simulink model "PhaseII_opalrt_NoProtection"  (Simulink 8.8)
settings: Solver=ode3  StartTime=0.0  StopTime=inf  FixedStep=Ts  RelTol=1e-5  EnableMultiTasking=on
PostLoadFcn:
  | %BESS ctrl
  | Kpf=0.005*3*12;
  | Kif=5*6;
  | 
  | Kpf1=0.005*3*12;
  | Kif1=5*6;
  | Kp_v=0.016*15*35;
  | Ki_v=12*25;
  | 
  | Kp_v1=0.016*15*35;
  | Ki_v1=12*25;
  | 
  | Vabc_B=12.47e3;
  | Vdc_ref=Vabc_B*2;
  | Kpwm=sqrt(2)*Vabc_B/Vdc_ref;
  | ZB=Vabc_B^2/1e6;
  | R=0.005*ZB;
  | Ibasefull=673/2*sqrt(2);
  | 
  | 
  | Ts_Control=1e-4;
  | ts=0.05;
  | delay=0.2;
  | offset=10e3;
  | t_plan=60;
  | t_monitor=.2;
  | t_mon=t_monitor;
  | scalingfactor=1;
  | x=0.5;
  | n=6;
  | %t_plan=1/15;
  | %t_monitor=10/900;
  | %t_mon=10/900;
  | 
  | %t_plan=1/5;
  | %t_monitor=10/300;
  | %t_mon=10/300;
  | %scalingfactor=1/300;
  | 
  | f0=60;
  | 
  | Pabc_B=1e6;
  | Iabc_B=Pabc_B*sqrt(2/3)/Vabc_B;  % pk value
  | Imax_1=2.5;
  | Ptrans_B=Pabc_B*200;
  | 
  | Vdc_ref=Vabc_B*2;
  | 
  | ZB=Vabc_B^2/Pabc_B;
  | L=0.1*ZB/2/pi/60;
  | R=0.1*ZB;
  | C=1/(4*pi^2*(2e3)^2*L);
  | 
  | LL=0.005*ZB/2/pi/60;
  | RR=0.005*ZB;
  | 
  | RC=0.02;
  | 
  | %%% Initial SOC %%%%
  | SOC_ini_BESS1=0.5;
  | ... (+223 lines)
InitFcn:
  | %BESS ctrl
  | Kpf=0.005*3*12;
  | Kif=5*6;
  | 
  | Kpf1=0.005*3*12;
  | Kif1=5*6;
  | Kp_v=0.016*15*35;
  | Ki_v=12*25;
  | 
  | Kp_v1=0.016*15*35;
  | Ki_v1=12*25;
  | 
  | Vabc_B=12.47e3;
  | Vdc_ref=Vabc_B*2;
  | Kpwm=sqrt(2)*Vabc_B/Vdc_ref;
  | ZB=Vabc_B^2/1e6;
  | R=0.005*ZB;
  | Ibasefull=673/2*sqrt(2);
  | 
  | 
  | Ts_Control=1e-4;
  | ts=0.05;
  | delay=0.2;
  | offset=10e3;
  | t_plan=60;
  | t_monitor=.2;
  | t_mon=t_monitor;
  | scalingfactor=1;
  | x=0.5;
  | n=6;
  | %t_plan=1/15;
  | %t_monitor=10/900;
  | %t_mon=10/900;
  | 
  | %t_plan=1/5;
  | %t_monitor=10/300;
  | %t_mon=10/300;
  | %scalingfactor=1/300;
  | 
  | f0=60;
  | 
  | Pabc_B=1e6;
  | Iabc_B=Pabc_B*sqrt(2/3)/Vabc_B;  % pk value
  | Imax_1=2.5;
  | Ptrans_B=Pabc_B*200;
  | 
  | Vdc_ref=Vabc_B*2;
  | 
  | ZB=Vabc_B^2/Pabc_B;
  | L=0.1*ZB/2/pi/60;
  | R=0.1*ZB;
  | C=1/(4*pi^2*(2e3)^2*L);
  | 
  | LL=0.005*ZB/2/pi/60;
  | RR=0.005*ZB;
  | 
  | RC=0.02;
  | 
  | %%% Initial SOC %%%%
  | SOC_ini_BESS1=0.5;
  | ... (+223 lines)
undefined symbols (not defined in the file): D1, Delta, DiscIntNeverNeededParam, Left, PG2ref, type, V
libraries: powerlib x220, powerlib_meascontrol x82, dspstat3 x54, dsparch4 x43, dspswit3 x24, simulink x19, simulink_extras x12, powerlib_extras x11, ssn_lib x7, artemis x6, rtlab x5, rtio_generic_dnp3 x5
(part 3 of 9)

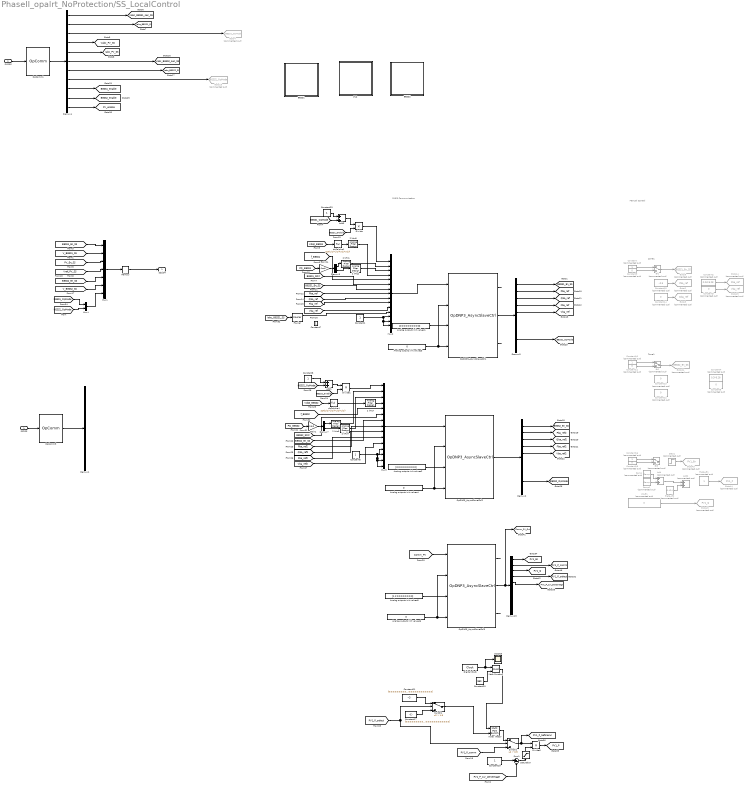
== system PhaseII_opalrt_NoProtection/SS_LocalControl ==
  note: DNP3 Communication
  note: Manual Control
  note: Zone1
  note: Zone1
  SC2SS : Inport
  SM2SS : Inport  Port=2
  2 kHz{1..5,7} (6 alike) : dsparch4/Analog Filter Design  method=Butterworth  filttype=Lowpass  N=2  Wlo=2*pi*5  Whi=80  Rp=2  Rs=40
  Add : Sum  Commented=on
  Add1 : Sum
  Add2 : Sum  Commented=on
  Add3 : Sum
  Analog outputs init values1 : Constant  Value=[0 0 0 0 0 0 0 0 0 0]
  Analog outputs init values2 : Constant  Value=[0 0 0 0 0 0 0 0 0 0]
  Analog outputs init values3 : Constant  Value=0
  Analog outputs init values4 : Constant  Value=0
  Analog outputs init values5 : Constant  Value=[1 2 0 0 0 0 0 0 0 0]
  Analog outputs init values6 : Constant  Value=0
  BESS1 : Subsystem
  BESS2 : Subsystem
  Br1 : ManualSwitch  Commented=on
  Br2 : ManualSwitch  Commented=on
  Br3 : ManualSwitch  Commented=on
  Constant : Constant  Commented=on
  Constant{1,6..8,19,23} (6 alike) : Constant
  Constant10 : Constant  Commented=on
  Constant{3,5,9,11..14,18} (8 alike) : Constant  Commented=on  Value=0
  Constant15 : Constant  Commented=on  Value=-0.5
  Constant16 : Constant  Commented=on
  Constant17 : Constant  Value=[0,0,0,0,0,0,0,0,0,0,0,0,0,0,0,0,0,0,0,0,0,0,0,0,0,0,0,0,0,0,0,0,0,0,0,0,0,0,0,0,0.00637590701003014,0.00637590701003014,0.00637590701003014,0.00637590701003014,0.00637590701003014,0.00637590701003014,0.00637590701003014,0.00637590701003014,0.00637590701003014,0.00637590701003014,0.00637590701003014,0.00637590701003014,0.00637590701003014,0.00637590701003014,0.00637590701003014,0.00637590701003014,0.00637590701003014,0.00637590701003014,0.00637590701003014,0.00637590701003014,0.0597883305113194,0.0597883305113194,0.0597883305113194,0.0597883305113194,0.0597883305113194,0.0597883305113194,0.0597883305113194,0.0597883305113194,0.0597883305113194,0.0597883305113194,0.0597883305113194,0.0597883305113194,0.0597883305113194,0.0597883305113194,0.0597883305113194,0.0597883305113194,0.0597883305113194,0.0597883305113194,0.0597883305113194,0.0597883305113194,0.191640198758314,0.191640198758314,0.191640198758314,0.191640198758314,0.191640198758314,0.191640198758314,0.191640198758314,0.191640198758314,0.191640198758314,0.191640198758314,0.191640198758314,0.191640198758314,0.191640198758314,0.191640198758314,0.191640198758314,0.191640198758314,0.191640198758314,0.191640198758314,0.191640198758314,0.191640198758314,0.258183655928258,0.258183655928258,0.258183655928258,0.258183655928258,0.258183655928258,0.258183655928258,0.258183655928258,0.258183655928258,0.258183655928258,0.258183655928258,0.258183655928258,0.258183655928258,0.258183655928258,0.258183655928258,0.258183655928258,0.258183655928258,0.258183655928258,0.258183655928258,0.258183655928258,0.258183655928258,0.318938480096502,0.318938480096502,0.318938480096502,0.318938480096502,0.318938480096502,0.318938480096502,0.318938480096502,0.318938480096502,0.318938480096502,0.318938480096502,0.318938480096502,0.318938480096502,0.318938480096502,0.318938480096502,0.318938480096502,0.318938480096502,0.318938480096502,0.318938480096502,0.318938480096502,0.318938480096502,0.451835046830676,0.451835046830676,0.451835046830676,0.451835046830676,0.451835046830676,0.451835046830676,0.451835046830676,0.451835046830676,0.451835046830676,0.451835046830676,0.451835046830676,0.451835046830676,0.451835046830676,0.451835046830676,0.451835046830676,0.451835046830676,0.451835046830676,0.451835046830676,0.451835046830676,0.451835046830676,0.659184087530387,0.659184087530387,0.659184087530387,0.659184087530387,0.659184087530387,0.659184087530387,0.659184087530387,0.659184087530387,0.659184087530387,0.659184087530387,0.659184087530387,0.659184087530387,0.659184087530387,0.659184087530387,0.659184087530387,0.659184087530387,0.659184087530387,0.659184087530387,0.659184087530387,0.659184087530387,0.827159209540989,0.827159209540989,0.827159209540989,0.827159209540989,0.827159209540989,0.827159209540989,0.827159209540989,0.827159209540989,0.827159209540989,0.827159209540989,0.827159209540989,0.827159209540989,0.827159209540989,0.827159209540989,0.827159209540989,0.827159209540989,0.827159209540989,0.827159209540989,0.827159209540989,0.827159209540989,1.02022332643508,1.02022332643508,1.02022332643508,1.02022332643508,1.02022332643508,1.02022332643508,1.02022332643508,1.02022332643508,1.02022332643508,1.02022332643508,1.02022332643508,1.02022332643508,1.02022332643508,1.02022332643508,1.02022332643508,1.02022332643508,1.02022332643508,1.02022332643508,1.02022332643508,1.02022332643508,1.18871489543793,1.18871489543793,1.18871489543793,1.18871489543793,1.18871489543793,1.18871489543793,1.18871489543793,1.18871489543793,1.18871489543793,1.18871489543793,1.18871489543793,1.18871489543793,1.18871489543793,1.18871489543793,1.18871489543793,1.18871489543793,1.18871489543793,1.18871489543793,1.18871489543793,1.18871489543793,1.35005293581671,1.35005293581671,1.35005293581671,1.35005293581671,1.35005293581671,1.35005293581671,1.35005293581671,1.35005293581671,1.35005293581671,1.35005293581671,1.35005293581671,1.35005293581671,1.35005293581671,1.35005293581671,1.35005293581671,1.35005293581671,1.35005293581671 ...(+10071 chars)]
  Constant2 : Constant  Commented=on  Value=0.04*6.28
  Constant20 : Constant  Value=960
  Constant21 : Constant  Value=[0,0,0,0,0,0,0,0,0,0,0,0,0,0,0,0,0,0,0,0,0,0,0,0,0,0,0,0,0,0,0,0,0,0,0,0,0,0,0,0,0,0,0,0,0,0,0,0,0,0,0,0,0,0,0,0,0,0,0,0,0.00981250996274463,0.00981250996274463,0.00981250996274463,0.00981250996274463,0.00981250996274463,0.00981250996274463,0.00981250996274463,0.00981250996274463,0.00981250996274463,0.00981250996274463,0.00981250996274463,0.00981250996274463,0.00981250996274463,0.00981250996274463,0.00981250996274463,0.00981250996274463,0.00981250996274463,0.00981250996274463,0.00981250996274463,0.00981250996274463,0.132748194010081,0.132748194010081,0.132748194010081,0.132748194010081,0.132748194010081,0.132748194010081,0.132748194010081,0.132748194010081,0.132748194010081,0.132748194010081,0.132748194010081,0.132748194010081,0.132748194010081,0.132748194010081,0.132748194010081,0.132748194010081,0.132748194010081,0.132748194010081,0.132748194010081,0.132748194010081,0.386564366030885,0.386564366030885,0.386564366030885,0.386564366030885,0.386564366030885,0.386564366030885,0.386564366030885,0.386564366030885,0.386564366030885,0.386564366030885,0.386564366030885,0.386564366030885,0.386564366030885,0.386564366030885,0.386564366030885,0.386564366030885,0.386564366030885,0.386564366030885,0.386564366030885,0.386564366030885,0.625701271422546,0.625701271422546,0.625701271422546,0.625701271422546,0.625701271422546,0.625701271422546,0.625701271422546,0.625701271422546,0.625701271422546,0.625701271422546,0.625701271422546,0.625701271422546,0.625701271422546,0.625701271422546,0.625701271422546,0.625701271422546,0.625701271422546,0.625701271422546,0.625701271422546,0.625701271422546,0.553924369190750,0.553924369190750,0.553924369190750,0.553924369190750,0.553924369190750,0.553924369190750,0.553924369190750,0.553924369190750,0.553924369190750,0.553924369190750,0.553924369190750,0.553924369190750,0.553924369190750,0.553924369190750,0.553924369190750,0.553924369190750,0.553924369190750,0.553924369190750,0.553924369190750,0.553924369190750,0.647873932663837,0.647873932663837,0.647873932663837,0.647873932663837,0.647873932663837,0.647873932663837,0.647873932663837,0.647873932663837,0.647873932663837,0.647873932663837,0.647873932663837,0.647873932663837,0.647873932663837,0.647873932663837,0.647873932663837,0.647873932663837,0.647873932663837,0.647873932663837,0.647873932663837,0.647873932663837,1.50320712211045,1.50320712211045,1.50320712211045,1.50320712211045,1.50320712211045,1.50320712211045,1.50320712211045,1.50320712211045,1.50320712211045,1.50320712211045,1.50320712211045,1.50320712211045,1.50320712211045,1.50320712211045,1.50320712211045,1.50320712211045,1.50320712211045,1.50320712211045,1.50320712211045,1.50320712211045,1.50449928127173,1.50449928127173,1.50449928127173,1.50449928127173,1.50449928127173,1.50449928127173,1.50449928127173,1.50449928127173,1.50449928127173,1.50449928127173,1.50449928127173,1.50449928127173,1.50449928127173,1.50449928127173,1.50449928127173,1.50449928127173,1.50449928127173,1.50449928127173,1.50449928127173,1.50449928127173,2,2,2,2,2,2,2,2,2,2,2,2,2,2,2,2,2,2,2,2,1.59623976041451,1.59623976041451,1.59623976041451,1.59623976041451,1.59623976041451,1.59623976041451,1.59623976041451,1.59623976041451,1.59623976041451,1.59623976041451,1.59623976041451,1.59623976041451,1.59623976041451,1.59623976041451,1.59623976041451,1.59623976041451,1.59623976041451,1.59623976041451,1.59623976041451,1.59623976041451,1.04765330636163,1.04765330636163,1.04765330636163,1.04765330636163,1.04765330636163,1.04765330636163,1.04765330636163,1.04765330636163,1.04765330636163,1.04765330636163,1.04765330636163,1.04765330636163,1.04765330636163,1.04765330636163,1.04765330636163,1.04765330636163,1.04765330636163,1.04765330636163,1.04765330636163,1.04765330636163,0.944545776431073,0.944545776431073,0.944545776431073,0.944545776431073,0.944545776431073,0.944545776431073,0.944545776431073,0.944545776431073,0.944545776431073,0.944545776431073,0.944545776431073,0.944545776431073,0.944545776431073,0.944545776431073,0.944545776431073 ...(+10070 chars)]
  Constant4 : Constant  Commented=on  Value=0.2*6.28
  Demux1 : Demux  Outputs=[1 1 1 1 1 1]
  Demux13 : Demux  Outputs=10
  Demux2 : Demux  Outputs=10
  Demux3 : Demux  Outputs=2
  Demux4 : Demux  Outputs=[3 3 1 3 3 3 3 1 1 1 1]
  Demux5 : Demux  Outputs=10
  Demux7 : Demux  Outputs=2
  Digital Clock : DigitalClock  SampleTime=[0,1]
  Divide : Product  Inputs=**
  Divide1 : Product  Inputs=**
  Divide6 : Product  Inputs=**
  Fourier : powerlib_meascontrol/Measurements/Fourier  Freq=60  n=1  InInit=[0, 0]  Ts=0
  Gain1 : Gain  Gain=-1e-6
  Gain24 : Gain  Gain=-1e-6
  Goto14 : Goto  Commented=on  GotoTag=Fba_ref  TagVisibility=global
  Goto15 : Goto  Commented=on  GotoTag=Vba_ref  TagVisibility=global
  Goto2 : Goto  Commented=on  GotoTag=Pba_ref  TagVisibility=global
  Goto23 : Goto  Commented=on  GotoTag=BESS2_OpMode  TagVisibility=global
  Goto24 : Goto  Commented=on  GotoTag=BESS2_En_SS  TagVisibility=global
  Goto3 : Goto  Commented=on  GotoTag=Qba_ref  TagVisibility=global
  Goto4 : Goto  Commented=on  GotoTag=BESS1_OpMode  TagVisibility=global
  Goto43 : Goto  Commented=on  GotoTag=PV1_En  TagVisibility=global
  Goto44 : Goto  Commented=on  GotoTag=PV1_P  TagVisibility=global
  Goto45 : Goto  Commented=on  GotoTag=PV1_Q  TagVisibility=global
  Goto9 : Goto  Commented=on  GotoTag=BESS1_En_SS  TagVisibility=global
  Index Vector : MultiPortSwitch  DataPortOrder=Zero-based contiguous  Inputs=1  zeroidx=on
  Math Function : Math  Operator=mod  SaturateOnIntegerOverflow=on
  Memory : Memory
  Mux1 : Mux  Inputs=[1 3 1 3 1 3 2]
  Mux2 : Mux  Inputs=15
  Mux3 : Mux  Inputs=15
  Mux4 : Mux  Inputs=2
  OpComm1 : rtlab/OpComm  nbport=1  groupe_acq=1  subsys_rate=0  st=0  Synchronization=on  Interpolation=on  Threshold=1.0  Missed_Data=off  Sim_Time=off  Samples=off  dynSigOut=off  from_console=0  warning_done=off  writeOpCommFile=off  Offset=off
  OpComm3 : rtlab/OpComm  nbport=1  groupe_acq=1  subsys_rate=0  st=0  Synchronization=on  Interpolation=on  Threshold=1.0  Missed_Data=off  Sim_Time=off  Samples=off  dynSigOut=off  from_console=1  warning_done=off  writeOpCommFile=off  Offset=off
  OpDNP3_AsyncSlaveCtrl1 : rtio_generic_dnp3/OpDNP3_AsyncSlaveCtrl  dev_id=3  nbr_aout=10  nbr_bout=1  cfg_name='AsyncDNP3_Slave_cfg.xml'  exe_name='AsyncDNP3_Slave'  nic_name='eth3'  link_addr_remote=7  link_addr_local=8  ip_addr_local='160.36.56.202'  tcp_port_local=18000  dnp3_options=0
  OpDNP3_AsyncSlaveCtrl2 : rtio_generic_dnp3/OpDNP3_AsyncSlaveCtrl  dev_id=4  nbr_aout=10  nbr_bout=1  cfg_name='AsyncDNP3_Slave_cfg.xml'  exe_name='AsyncDNP3_Slave'  nic_name='eth3'  link_addr_remote=9  link_addr_local=10  ip_addr_local='160.36.56.207'  tcp_port_local=18000  dnp3_options=0
  OpDNP3_AsyncSlaveCtrl3 : rtio_generic_dnp3/OpDNP3_AsyncSlaveCtrl  dev_id=2  nbr_aout=10  nbr_bout=1  cfg_name='AsyncDNP3_Slave_cfg.xml'  exe_name='AsyncDNP3_Slave'  nic_name='eth3'  link_addr_remote=5  link_addr_local=6  ip_addr_local='160.36.56.201'  tcp_port_local=18000  dnp3_options=0
  PV2 : Subsystem
  Ramp : simulink/Sources/Ramp  Commented=on  slope=0.5  start=0.5  X0=0
  Ramp1 : simulink/Sources/Ramp  Commented=on  slope=-0.5  start=2.762  X0=0
  Saturation : Saturate  UpperLimit=1  LowerLimit=0
  Scope3 : Scope
  Step1 : Step  Commented=on  SampleTime=0
  Sum1 : Sum  Inputs=|+-
  Switch1 : Switch  Criteria=u2 > Threshold  Threshold=1.5
  Switch2 : Switch  Criteria=u2 > Threshold  Threshold=0.5
  Vd_G1 : Constant  Commented=on  Value=0
  dq2alpha1 : Fcn  Expr=sqrt(u(1)*u(1)+u(2)*u(2))
  dq2alpha4 : Fcn  Expr=sqrt(u(1)*u(1)+u(2)*u(2))
  theta_G1 : Constant  Commented=on
  theta_G2 : Constant  Commented=on  Value=0.424
  "SS2SM " : Outport
  tag scope: BESS1_En_SS=global, BESS1_OpMode=global, BESS1_enable=global, BESS2_En_SS=global, BESS2_OpMode=global, BESS2_enable=global, Comm_PV_Out=global, Fba_ref2=global, Fba_ref=global, Iabc_BESS1_SS=global, Iabc_BESS2_SS=global, Iabc_PV_SS=global, PV1_En=global, PV1_P=global, PV1_P_beforecur=global, PV1_P_comm=global, PV1_P_cur_percentage=global, PV1_P_select=global, PV1_Q=global, PV_enable=global, Pba_ref2=global, Pba_ref=global, Qba_ref2=global, Qba_ref=global, Vabc_BESS1_sec_SS=global, Vabc_BESS2_sec_SS=global, Vabc_PV_SS=global, Vba_ref2=global, Vba_ref=global
  wires:
  SC2SS/1 -> OpComm3/1
  SM2SS/1 -> OpComm1/1
  OpComm1/1 -> Demux4/1
  Demux4/1 -> [Vabc_BESS1_sec_SS]
  Demux4/2 -> [Iabc_BESS1_SS]
  Memory/1 -> "SS2SM "/1
  Mux1/1 -> Memory/1
  [BESS1_En_SS] -> Mux1/1
  [V_BESS1_SS] -> Mux1/2
  OpComm3/1 -> Demux1/1
  Demux4/4 -> [Vabc_PV_SS]
  Demux4/5 -> [Iabc_PV_SS]
  [PV_En_SS] -> Mux1/3
  [Vref_PV_SS] -> Mux1/4
  Constant2/1 -> Goto14/1
  Constant3/1 -> Goto15/1
  [BESS2_En_SS] -> Mux1/5
  [V_BESS2_SS] -> Mux1/6
  Demux4/6 -> [Vabc_BESS2_sec_SS]
  Demux4/7 -> [Iabc_BESS2_SS]
  Demux4/9 -> [BESS1_enable]
  Demux4/10 -> [BESS2_enable]
  Demux4/3 -> Goto4/1
  [BESS1_OpMode] -> Add3/2
  Constant23/1 -> Add3/1
  Add3/1 -> Divide/1
  [BESS1_enable] -> Divide/2
  [Vdq0_BESS1] -> dq2alpha1/1
  Demux3/1 -> 2 kHz1/1
  Demux3/2 -> 2 kHz2/1
  [PQ_BESS1] -> Gain24/1
  Divide/1 -> Mux2/1
  [BESS1_SOC] -> Mux2/6
  Constant1/1 -> Mux2/15, Mux2/14, Mux2/13
  Analog outputs init values3/1 -> OpDNP3_AsyncSlaveCtrl1/2, OpDNP3_AsyncSlaveCtrl1/4
  OpDNP3_AsyncSlaveCtrl1/2 -> Demux5/1
  OpDNP3_AsyncSlaveCtrl1/3 -> ?
  OpDNP3_AsyncSlaveCtrl1/1 -> ?
  Mux2/1 -> OpDNP3_AsyncSlaveCtrl1/1
  Analog outputs init values1/1 -> OpDNP3_AsyncSlaveCtrl1/3
  Demux5/1 -> [BESS1_En_SS]
  Demux5/2 -> [Pba_ref]
  Demux5/3 -> [Qba_ref]
  Demux5/4 -> [Fba_ref]
  Demux5/5 -> [Vba_ref]
  [BESS1_En_SS] -> Mux2/7
  [Pba_ref] -> Mux2/8
  [Qba_ref] -> Mux2/9
  [Fba_ref] -> Mux2/10
  [Vba_ref] -> Mux2/11
  [Iabc_BESS1_SS] -> Fourier/1
  Fourier/1 -> Mux2/12
  Demux4/11 -> [PV_enable]
  [BESS2_OpMode] -> Add1/2
  Constant8/1 -> Add1/1
  Add1/1 -> Divide1/1
  [BESS2_enable] -> Divide1/2
  [Vdq0_BESS2] -> dq2alpha4/1
  Demux7/1 -> 2 kHz3/1
  Demux7/2 -> 2 kHz4/1
  [PQ_BESS2] -> Gain1/1
  Divide1/1 -> Mux3/1
  [BESS2_SOC] -> Mux3/6
  [BESS2_En_SS] -> Mux3/7
  [Pba_ref2] -> Mux3/8
  [Qba_ref2] -> Mux3/9
  [Fba_ref2] -> Mux3/10
  [Vba_ref2] -> Mux3/11
  Constant6/1 -> Mux3/12, Mux3/13, Mux3/14, Mux3/15
  Analog outputs init values4/1 -> OpDNP3_AsyncSlaveCtrl2/4, OpDNP3_AsyncSlaveCtrl2/2
  Analog outputs init values2/1 -> OpDNP3_AsyncSlaveCtrl2/3
  Mux3/1 -> OpDNP3_AsyncSlaveCtrl2/1
  OpDNP3_AsyncSlaveCtrl2/2 -> Demux2/1
  Demux2/1 -> [BESS2_En_SS]
  Demux2/2 -> [Pba_ref2]
  Demux2/3 -> [Qba_ref2]
  Demux2/4 -> [Fba_ref2]
  Demux2/5 -> [Vba_ref2]
  Constant/1 -> Br1/1
  Constant9/1 -> Br1/2
  Constant10/1 -> Br2/1
  Constant11/1 -> Br2/2
  Constant15/1 -> Goto2/1
  Constant14/1 -> Goto3/1
  Analog outputs init values6/1 -> OpDNP3_AsyncSlaveCtrl3/4, OpDNP3_AsyncSlaveCtrl3/2
  OpDNP3_AsyncSlaveCtrl3/2 -> Demux13/1, [Comm_PV_Out]
  OpDNP3_AsyncSlaveCtrl3/3 -> ?
  OpDNP3_AsyncSlaveCtrl3/1 -> ?
  [Comm_PV] -> OpDNP3_AsyncSlaveCtrl3/1
  Demux13/1 -> [PV1_En]
  Demux13/3 -> [PV1_Q]
  Constant16/1 -> Br3/1
  Constant18/1 -> Br3/2
  Vd_G1/1 -> Goto45/1
  Demux13/2 -> [PV1_P_comm]
  Constant20/1 -> Math Function/2
  Math Function/1 -> Index Vector/1
  Constant21/1 -> Switch1/1
  Switch1/1 -> Index Vector/2
  Demux13/4 -> [PV1_P_select]
  Constant17/1 -> Switch1/3
  [PV1_P_select] -> Switch1/2, Switch2/2
  [PV1_P_comm] -> Switch2/3
  Index Vector/1 -> Switch2/1
  Digital Clock/1 -> Scope3/1, Math Function/1
  Demux13/5 -> [PV1_P_cur_percentage]
  Switch2/1 -> [PV1_P_beforecur], Divide6/1
  Divide6/1 -> [PV1_P]
  Constant19/1 -> Sum1/1
  [PV1_P_cur_percentage] -> Sum1/2
  Sum1/1 -> Saturation/1
  Saturation/1 -> Divide6/2
  Analog outputs init values5/1 -> OpDNP3_AsyncSlaveCtrl3/3
  Step1/1 -> Goto43/1
  Ramp/1 -> Add/1
  Ramp1/1 -> Add/2
  Add/1 -> Add2/1
  theta_G2/1 -> Add2/2
  theta_G1/1 -> Goto44/1
  Gain24/1 -> Demux3/1
  Gain1/1 -> Demux7/1
  2 kHz1/1 -> Mux2/2
  2 kHz2/1 -> Mux2/3
  dq2alpha1/1 -> 2 kHz5/1
  [f_BESS1] -> Mux2/5
  dq2alpha4/1 -> 2 kHz7/1
  [f_BESS2] -> Mux3/5
  2 kHz3/1 -> Mux3/2
  2 kHz4/1 -> Mux3/3
  [BESS1_OpMode] -> Mux4/1
  [BESS2_OpMode] -> Mux4/2
  Mux4/1 -> Mux1/7
  Br1/1 -> Goto9/1
  Br2/1 -> Goto24/1
  Demux5/9 -> [BESS1_OpMode]
  Demux2/9 -> [BESS2_OpMode]
  Demux4/8 -> Goto23/1
  2 kHz5/1 -> Mux2/4
  2 kHz7/1 -> Mux3/4

== system PhaseII_opalrt_NoProtection/SM_System/Battery 2 ==
  Demux2 : Demux  Outputs=3
  Gain2 : Gain
  Gain3 : Gain  Gain=Vdc_ref/2
  Gain5 : Gain  Gain=480
  vsa : powerlib/Electrical Sources/Controlled Voltage Source  Initialize=on  Source_Type=AC  Amplitude=0  Phase=0  Frequency=0  Measurements=None
  vsb : powerlib/Electrical Sources/Controlled Voltage Source  Initialize=on  Source_Type=AC  Amplitude=0  Phase=0  Frequency=0  Measurements=None
  vsc : powerlib/Electrical Sources/Controlled Voltage Source  Initialize=on  Source_Type=AC  Amplitude=0  Phase=0  Frequency=0  Measurements=None
  A : PMIOPort  Tag=PMCPort  Port=1  Side=Right
  B : PMIOPort  Tag=PMCPort  Port=2  Side=Right
  C : PMIOPort  Tag=PMCPort  Port=3  Side=Right
  wires:
  Demux2/1 -> vsa/1
  Demux2/2 -> vsb/1
  Demux2/3 -> vsc/1
  [V_BESS2] -> Gain5/1
  Gain5/1 -> Demux2/1
  connections:
  vsc/RConn1 -- C/RConn1
  vsc/LConn1 -- vsb/LConn1 -- vsa/LConn1
  B/RConn1 -- vsb/RConn1
  vsa/RConn1 -- A/RConn1

== system PhaseII_opalrt_NoProtection/SM_System/Battery 1  ==
  Demux2 : Demux  Outputs=3
  Gain2 : Gain
  Gain3 : Gain  Gain=Vdc_ref/2
  Gain5 : Gain  Gain=480
  vsa : powerlib/Electrical Sources/Controlled Voltage Source  Initialize=on  Source_Type=AC  Amplitude=0  Phase=0  Frequency=0  Measurements=None
  vsb : powerlib/Electrical Sources/Controlled Voltage Source  Initialize=on  Source_Type=AC  Amplitude=0  Phase=0  Frequency=0  Measurements=None
  vsc : powerlib/Electrical Sources/Controlled Voltage Source  Initialize=on  Source_Type=AC  Amplitude=0  Phase=0  Frequency=0  Measurements=None
  A : PMIOPort  Tag=PMCPort  Port=1  Side=Right
  B : PMIOPort  Tag=PMCPort  Port=2  Side=Right
  C : PMIOPort  Tag=PMCPort  Port=3  Side=Right
  wires:
  Demux2/1 -> vsa/1
  Demux2/2 -> vsb/1
  Demux2/3 -> vsc/1
  [V_BESS1] -> Gain5/1
  Gain5/1 -> Demux2/1
  connections:
  vsc/RConn1 -- C/RConn1
  vsc/LConn1 -- vsb/LConn1 -- vsa/LConn1
  B/RConn1 -- vsb/RConn1
  vsa/RConn1 -- A/RConn1

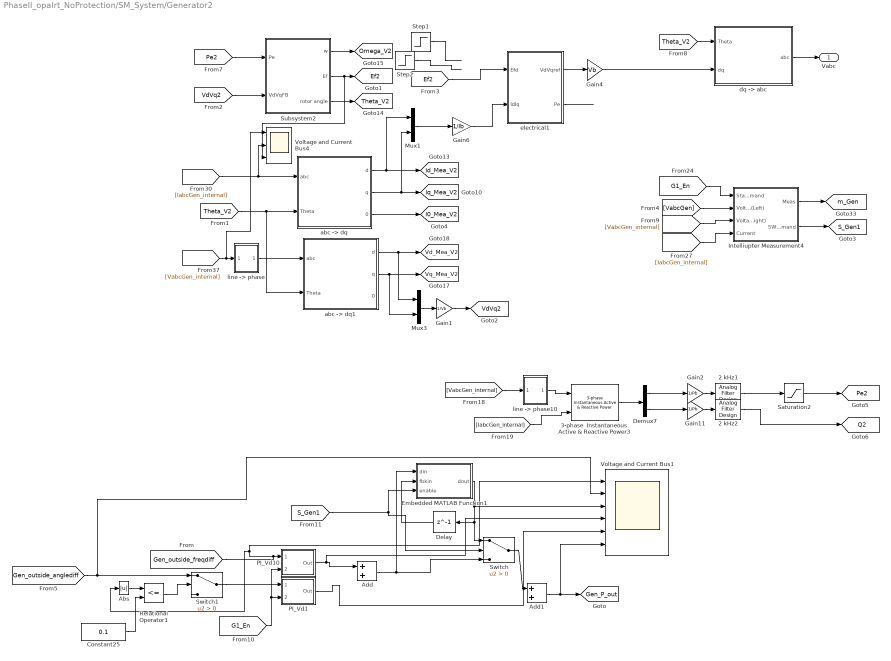
== system PhaseII_opalrt_NoProtection/SM_System/Generator2 ==
  2 kHz1 : dsparch4/Analog Filter Design  method=Butterworth  filttype=Lowpass  N=2  Wlo=2*pi*5  Whi=80  Rp=2  Rs=40
  2 kHz2 : dsparch4/Analog Filter Design  method=Butterworth  filttype=Lowpass  N=2  Wlo=2*pi*5  Whi=80  Rp=2  Rs=40
  3-phase  Instantaneous  Active & Reactive Power3 : powerlib_extras/Measurements/3-phase  Instantaneous  Active & Reactive Power
  Abs : Abs
  Add : Sum
  Add1 : Sum
  Constant25 : Constant  Value=0.1
  Delay : Delay  DelayLength=1  InitialCondition=0
  Demux7 : Demux  Outputs=2
  Embedded MATLAB Function1 : MATLAB Function  TreatAsAtomicUnit=on
  Gain1 : Gain  Gain=1/Vb
  Gain11 : Gain  Gain=1/Pb
  Gain2 : Gain  Gain=1/Pb
  Gain4 : Gain  Gain=Vb
  Gain6 : Gain  Gain=1/Ib
  Intelliupter Measurement4 : Subsystem
  Mux1 : Mux  Inputs=2
  Mux3 : Mux  Inputs=2
  PI_Vd1 : Subsystem
  PI_Vd10 : Subsystem
  Relational Operator1 : RelationalOperator  Operator=<=  OutDataTypeStr=boolean  RndMeth=Simplest
  Saturation2 : Saturate  UpperLimit=2  LowerLimit=-1  ZeroCross=off
  Step1 : Step  Before=1  SampleTime=0
  Step2 : Step  Time=22  After=0  SampleTime=0
  Subsystem2 : Subsystem
  Switch : Switch  Criteria=u2 > Threshold
  Switch1 : Switch  Criteria=u2 > Threshold
  Voltage and Current Bus1 : Scope  NumInputPorts=6
  Voltage and Current Bus4 : Scope  NumInputPorts=3
  "abc -> dq" : Subsystem
  "abc -> dq1" : Subsystem
  "dq -> abc" : Subsystem
  electrical1 : Subsystem
  "line -> phase" : Subsystem
  "line -> phase10" : Subsystem
  Vabc : Outport
  tag scope: Ef2=global, Gen_P_out=global, I0_Mea_V2=global, Id_Mea_V2=global, Iq_Mea_V2=global, Omega_V2=global, Pe2=global, Q2=global, S_Gen1=global, Theta_V2=global, VdVq2=global, Vd_Mea_V2=global, Vq_Mea_V2=global, m_Gen=global
  wires:
  "dq -> abc"/1(abc) -> Vabc/1
  "abc -> dq"/1(d) -> [Id_Mea_V2], Mux1/1
  "abc -> dq1"/1(d) -> [Vd_Mea_V2], Mux3/1
  "abc -> dq1"/2(q) -> [Vq_Mea_V2], Mux3/2
  [Theta_V2] -> "abc -> dq"/2(Theta), "abc -> dq1"/2(Theta)
  "line -> phase"/1(Vph) -> "abc -> dq1"/1(abc)
  Subsystem2/2(Ef) -> Voltage and Current Bus4/3, [Ef2]
  Subsystem2/3(rotor angle) -> [Theta_V2]
  [Pe2] -> Subsystem2/1(Pe)
  [VdVq2] -> Subsystem2/2(VdVqFB)
  Subsystem2/1(w) -> [Omega_V2]
  electrical1/2(Pe) -> ?
  electrical1/1(VdVqref) -> Gain4/1
  Mux1/1 -> Gain6/1
  "abc -> dq"/2(q) -> [Iq_Mea_V2], Mux1/2
  "abc -> dq"/3(0) -> [I0_Mea_V2]
  [Theta_V2] -> "dq -> abc"/1(Theta)
  Gain6/1 -> electrical1/2(IdIq)
  Gain4/1 -> "dq -> abc"/2(dq)
  Mux3/1 -> Gain1/1
  Gain1/1 -> [VdVq2]
  [IabcGen_internal] -> Voltage and Current Bus4/2, "abc -> dq"/1(abc)
  [VabcGen_internal] -> Voltage and Current Bus4/1, "line -> phase"/1(Vll)
  [VabcGen_internal] -> "line -> phase10"/1(Vll)
  "line -> phase10"/1(Vph) -> 3-phase  Instantaneous  Active & Reactive Power3/1
  [IabcGen_internal] -> 3-phase  Instantaneous  Active & Reactive Power3/2
  3-phase  Instantaneous  Active & Reactive Power3/1 -> Demux7/1
  Demux7/1 -> Gain2/1
  Gain2/1 -> 2 kHz1/1
  Demux7/2 -> Gain11/1
  Gain11/1 -> 2 kHz2/1
  [VabcGen_internal] -> Intelliupter Measurement4/3(Voltage (Right))
  [VabcGen] -> Intelliupter Measurement4/2(Voltage (Left))
  Intelliupter Measurement4/2(SW Command) -> [S_Gen1]
  Intelliupter Measurement4/1(Meas) -> [m_Gen]
  [IabcGen_internal] -> Intelliupter Measurement4/4(Current)
  [G1_En] -> Intelliupter Measurement4/1(Status command)
  [Gen_outside_freqdiff] -> Abs/1, Voltage and Current Bus1/1, PI_Vd10/1(Error)
  [Gen_outside_anglediff] -> Switch1/1, Voltage and Current Bus1/2
  PI_Vd10/1(Out) -> Voltage and Current Bus1/4, Add/1
  PI_Vd1/1(Out) -> Voltage and Current Bus1/5
  Add1/1 -> Voltage and Current Bus1/6, [Gen_P_out]
  [G1_En] -> PI_Vd10/2("Reset "), PI_Vd1/2("Reset ")
  [S_Gen1] -> Switch/2, Embedded MATLAB Function1/3(enable)
  Add/1 -> Embedded MATLAB Function1/1(din), Switch/3
  Switch/1 -> Add1/1
  Embedded MATLAB Function1/1(dout) -> Switch/1, Delay/1, Voltage and Current Bus1/3
  Delay/1 -> Embedded MATLAB Function1/2(fbkin)
  ? -> ?
  Switch1/1 -> PI_Vd1/1(Error)
  Relational Operator1/1 -> Switch1/2
  Constant25/1 -> Relational Operator1/2
  Abs/1 -> Relational Operator1/1
  2 kHz1/1 -> Saturation2/1
  2 kHz2/1 -> [Q2]
  [Ef2] -> electrical1/1(Efd)
  Step2/1 -> ?
  Step1/1 -> ?
  Saturation2/1 -> [Pe2]

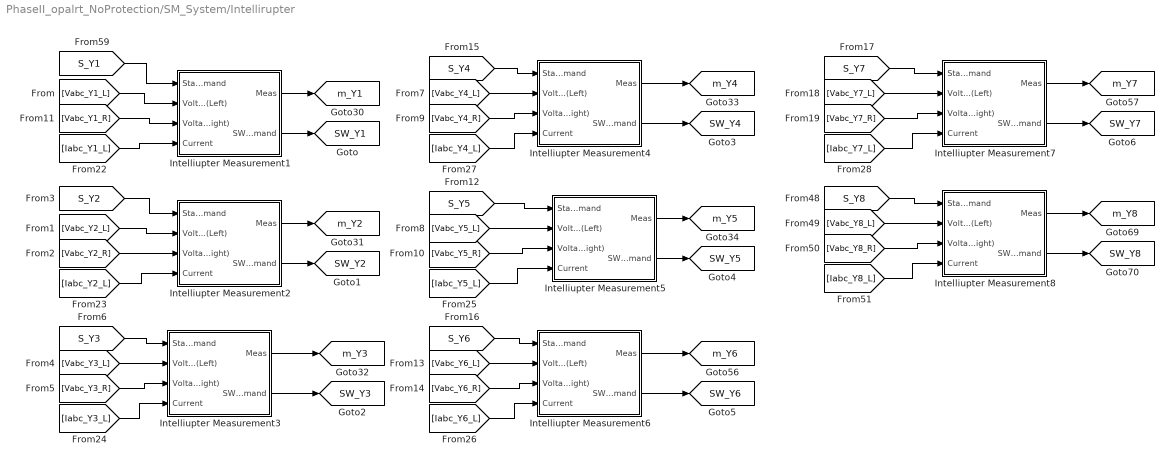
== system PhaseII_opalrt_NoProtection/SM_System/Intellirupter ==
  Intelliupter Measurement1 : Subsystem
  Intelliupter Measurement2 : Subsystem
  Intelliupter Measurement3 : Subsystem
  Intelliupter Measurement4 : Subsystem
  Intelliupter Measurement5 : Subsystem
  Intelliupter Measurement6 : Subsystem
  Intelliupter Measurement7 : Subsystem
  Intelliupter Measurement8 : Subsystem
  tag scope: SW_Y1=global, SW_Y2=global, SW_Y3=global, SW_Y4=global, SW_Y5=global, SW_Y6=global, SW_Y7=global, SW_Y8=global, m_Y1=global, m_Y2=global, m_Y3=global, m_Y4=global, m_Y5=global, m_Y6=global, m_Y7=global, m_Y8=global
  wires:
  Intelliupter Measurement1/2(SW Command) -> [SW_Y1]
  [Vabc_Y1_L] -> Intelliupter Measurement1/2(Voltage (Left))
  [S_Y1] -> Intelliupter Measurement1/1(Status command)
  [Vabc_Y1_R] -> Intelliupter Measurement1/3(Voltage (Right))
  [Vabc_Y2_R] -> Intelliupter Measurement2/3(Voltage (Right))
  [S_Y2] -> Intelliupter Measurement2/1(Status command)
  [Vabc_Y2_L] -> Intelliupter Measurement2/2(Voltage (Left))
  Intelliupter Measurement2/2(SW Command) -> [SW_Y2]
  Intelliupter Measurement3/2(SW Command) -> [SW_Y3]
  [Vabc_Y3_L] -> Intelliupter Measurement3/2(Voltage (Left))
  [S_Y3] -> Intelliupter Measurement3/1(Status command)
  [Vabc_Y3_R] -> Intelliupter Measurement3/3(Voltage (Right))
  [Vabc_Y6_R] -> Intelliupter Measurement6/3(Voltage (Right))
  [S_Y6] -> Intelliupter Measurement6/1(Status command)
  [Vabc_Y6_L] -> Intelliupter Measurement6/2(Voltage (Left))
  Intelliupter Measurement6/2(SW Command) -> [SW_Y6]
  Intelliupter Measurement5/2(SW Command) -> [SW_Y5]
  [Vabc_Y5_L] -> Intelliupter Measurement5/2(Voltage (Left))
  [S_Y5] -> Intelliupter Measurement5/1(Status command)
  [Vabc_Y5_R] -> Intelliupter Measurement5/3(Voltage (Right))
  [Vabc_Y4_R] -> Intelliupter Measurement4/3(Voltage (Right))
  [S_Y4] -> Intelliupter Measurement4/1(Status command)
  [Vabc_Y4_L] -> Intelliupter Measurement4/2(Voltage (Left))
  Intelliupter Measurement4/2(SW Command) -> [SW_Y4]
  Intelliupter Measurement7/2(SW Command) -> [SW_Y7]
  [Vabc_Y7_L] -> Intelliupter Measurement7/2(Voltage (Left))
  [S_Y7] -> Intelliupter Measurement7/1(Status command)
  [Vabc_Y7_R] -> Intelliupter Measurement7/3(Voltage (Right))
  [Iabc_Y1_L] -> Intelliupter Measurement1/4(Current)
  Intelliupter Measurement1/1(Meas) -> [m_Y1]
  [Iabc_Y2_L] -> Intelliupter Measurement2/4(Current)
  [Iabc_Y3_L] -> Intelliupter Measurement3/4(Current)
  [Iabc_Y7_L] -> Intelliupter Measurement7/4(Current)
  Intelliupter Measurement2/1(Meas) -> [m_Y2]
  Intelliupter Measurement3/1(Meas) -> [m_Y3]
  Intelliupter Measurement4/1(Meas) -> [m_Y4]
  Intelliupter Measurement5/1(Meas) -> [m_Y5]
  Intelliupter Measurement6/1(Meas) -> [m_Y6]
  Intelliupter Measurement7/1(Meas) -> [m_Y7]
  [Iabc_Y4_L] -> Intelliupter Measurement4/4(Current)
  [Iabc_Y5_L] -> Intelliupter Measurement5/4(Current)
  [Iabc_Y6_L] -> Intelliupter Measurement6/4(Current)
  Intelliupter Measurement8/2(SW Command) -> [SW_Y8]
  [Vabc_Y8_L] -> Intelliupter Measurement8/2(Voltage (Left))
  [S_Y8] -> Intelliupter Measurement8/1(Status command)
  [Vabc_Y8_R] -> Intelliupter Measurement8/3(Voltage (Right))
  [Iabc_Y8_L] -> Intelliupter Measurement8/4(Current)
  Intelliupter Measurement8/1(Meas) -> [m_Y8]
